simulink model "SIMU_CORRECTION_MODELE_ETAT"  (R2020a)
settings: Solver=VariableStepAuto  StartTime=0.0  StopTime=100  RelTol=1e-3
values from neighbouring files (symbols this model uses):
  Ki = Kcorr    (= 0.91078)    [identificat.m]    (also in projet.mat)
  KK = [8.92919305691  3.48652443238; 3.48652443238  3.11318497544]    [projet.mat]
  Kp = 5.8*Kcorr    (= 5.282524)    [identificat.m]    (also in projet.mat)
  Te = 0.005    [identificat.m]    (also in projet.mat)
libraries: cstblocks x3, simulink x1
settings Model: Creator=soual  LastModifiedBy=soual

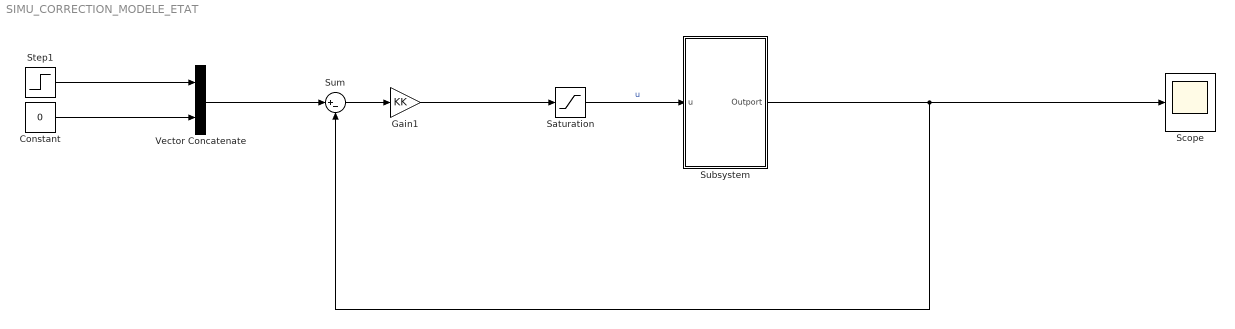
== system SIMU_CORRECTION_MODELE_ETAT ==
  Constant : Constant  Value=0
  Gain1 : Gain  Gain=KK
  Saturation : Saturate  UpperLimit=+9  LowerLimit=-9
  Scope : Scope
  Step1 : Step  Time=0  After=0  SampleTime=Te
  Subsystem : Subsystem
  Sum : Sum  Inputs=|+-
  Vector Concatenate : Concatenate
  wires:
  Saturation/1 -> Subsystem/1(u)  "u"
  Step1/1 -> Vector Concatenate/1
  Constant/1 -> Vector Concatenate/2
  Vector Concatenate/1 -> Sum/1
  Gain1/1 -> Saturation/1
  Sum/1 -> Gain1/1
  Subsystem/1(Outport) -> Sum/2, Scope/1

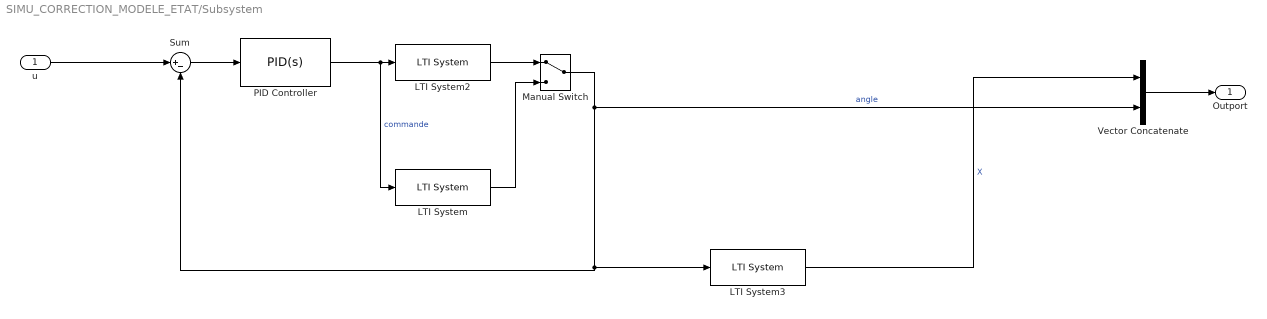
== system SIMU_CORRECTION_MODELE_ETAT/Subsystem ==
  u : Inport
  LTI System : cstblocks/LTI System  sys=tf_ordre2  IC=[]
  LTI System2 : cstblocks/LTI System  sys=G  IC=[]
  LTI System3 : cstblocks/LTI System  sys=sys  IC=[10; 0]
  Manual Switch : ManualSwitch
  PID Controller : simulink/Continuous/PID Controller  Controller=PID  Form=Parallel  TimeDomain=Continuous-time  UseExternalTs=off  SampleTime=Te  IntegratorMethod=Forward Euler  FilterMethod=Forward Euler  ControllerParametersSource=internal  P=Kp  I=Ki  D=0  UseFilter=on  N=100  TunerSelectOption=Transfer Function Based (PID Tuner App)  InitialConditionSource=internal  InitialConditionForIntegrator=0  InitialConditionForFilter=0  DifferentiatorICPrevScaledInput=0  ExternalReset=none  TrackingMode=off  Kt=1  LimitOutput=on  UpperSaturationLimit=+10  LowerSaturationLimit=-10  LinearizeAsGain=on  AntiWindupMode=none  Kb=1  POutMin=[]  POutMax=[]  IOutMin=[]  IOutMax=[]  DOutMin=[]  DOutMax=[]  NOutMin=[]  NOutMax=[]  SumOutMin=[]  SumOutMax=[]  SaturationOutMin=[]  SaturationOutMax=[]  PParamMin=[]  PParamMax=[]  IParamMin=[]  IParamMax=[]  DParamMin=[]  DParamMax=[]  NParamMin=[]  NParamMax=[]  KbParamMin=[]  KbParamMax=[]  KtParamMin=[]  KtParamMax=[]  KbOutMin=[]  KbOutMax=[]  KtOutMin=[]  KtOutMax=[]  IntegratorOutMin=[]  IntegratorOutMax=[]  FilterOutMin=[]  FilterOutMax=[]  SumI1OutMin=[]  SumI1OutMax=[]  SumI2OutMin=[]  SumI2OutMax=[]  SumI3OutMin=[]  SumI3OutMax=[]  SumI4OutMin=[]  SumI4OutMax=[]  SumDOutMin=[]  SumDOutMax=[]  DifferentiatorOutMin=[]  DifferentiatorOutMax=[]  FilterDiffOutCoefMin=[]  FilterDiffOutCoefMax=[]  ReciprocalOutMin=[]  ReciprocalOutMax=[]  SumDenOutMin=[]  SumDenOutMax=[]  SumNumOutMin=[]  SumNumOutMax=[]  DivideOutMin=[]  DivideOutMax=[]  UdiffTsProdOutMin=[]  UdiffTsProdOutMax=[]  NTsProdOutMin=[]  NTsProdOutMax=[]  UintegralTsProdOutMin=[]  UintegralTsProdOutMax=[]  UngainTsProdOutMin=[]  UngainTsProdOutMax=[]  IntegratorContinuousStateAttributes=''  IntegratorStateMustResolveToSignalObject=off  IntegratorRTWStateStorageClass=Auto  FilterContinuousStateAttributes=''  FilterStateMustResolveToSignalObject=off  FilterRTWStateStorageClass=Auto  ParallelPVariant=InternalParameters  IdealPVariant=Disabled  IVariant=InternalParameters  DVariant=InternalParameters  IntegratorVariant=Continuous  SatVariant=Enabled  AWVariant=Passthrough  PCopyVariant=Disabled  TRVariant=Disabled  FdbkBlocksVariant=Forward  IdealPFdbkVariant=Disabled  SatFdbkVariant=Disabled  DerivativeFilterVariant=ContFilter  NVariant=InternalParameters  NCopyVariant=Disabled  FilterICVariant=InternalICsFilter  IntegratorICVariant=InternalICs  ExternalResetVariant=Disabled  TRSumVariant=Passthrough  SumFdbkVariant=Disabled  SumVariant=Sum_PID  TsampFilterVariant=InternalTs  TsampNgainVariant=Passthrough  TsampIntegralVariant=Passthrough
  Sum : Sum  Inputs=|+-
  Vector Concatenate : Concatenate
  Outport : Outport
  wires:
  Sum/1 -> PID Controller/1
  Manual Switch/1 -> Vector Concatenate/2, Sum/2, LTI System3/1  "angle"
  PID Controller/1 -> LTI System/1, LTI System2/1  "commande"
  LTI System/1 -> Manual Switch/2
  LTI System2/1 -> Manual Switch/1
  u/1 -> Sum/1
  Vector Concatenate/1 -> Outport/1
  LTI System3/1 -> Vector Concatenate/1  "X"
